simulink model "Consigna_de_torque"  (R2023b)
settings: Solver=VariableStepAuto  StartTime=0.0  StopTime=10.0  RelTol=1e-3
values from neighbouring files (symbols this model uses):
  b_eq = b_m + b_l/(r^2)    (= 2.40277777778e-05)    [definicion_cte.m]
  k_l = m*l_cm + m_l*l_l    (= 1)    [definicion_cte.m]
  L_d = 6.6e-3    (= 0.0066)    [definicion_cte.m]
  L_q = 5.8e-3    (= 0.0058)    [definicion_cte.m]
  lambda_m = 0.016    [definicion_cte.m]
  P_p = 3    [definicion_cte.m]
  r = 120    [definicion_cte.m]
settings Model: Creator=MSI  LastModifiedBy=MSI

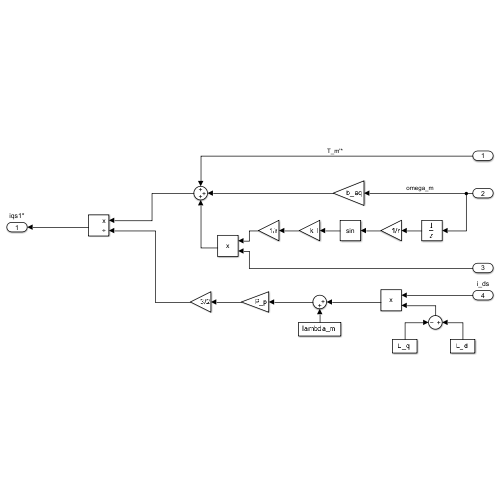
[thumbnail: Simulink's stored preview of the top-level diagram]
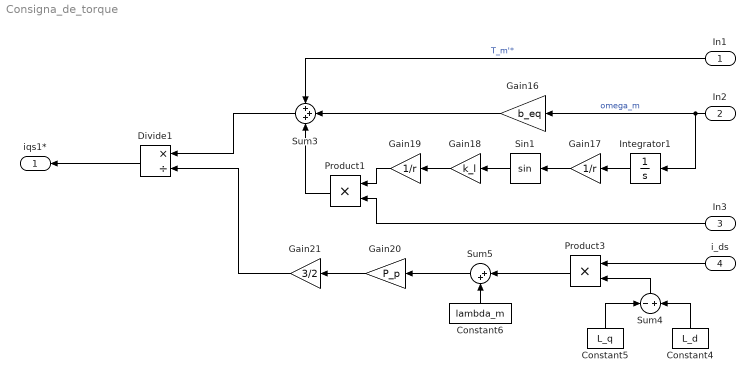
== system Consigna_de_torque ==
  In1 : Inport
  In2 : Inport  Port=2
  In3 : Inport  Port=3
  i_ds : Inport  Port=4
  Constant4 : Constant  Value=L_d
  Constant5 : Constant  Value=L_q
  Constant6 : Constant  Value=lambda_m
  Divide1 : Product  Inputs=*/
  Gain16 : Gain  Gain=b_eq
  Gain17 : Gain  Gain=1/r
  Gain18 : Gain  Gain=k_l
  Gain19 : Gain  Gain=1/r
  Gain20 : Gain  Gain=P_p
  Gain21 : Gain  Gain=3/2
  Integrator1 : Integrator
  Product1 : Product
  Product3 : Product
  Sin1 : Trigonometry
  Sum3 : Sum  Inputs=+++
  Sum4 : Sum  Inputs=-+
  Sum5 : Sum  Inputs=|++
  iqs1* : Outport
  wires:
  Gain16/1 -> Sum3/2
  In3/1 -> Product1/2
  Constant5/1 -> Sum4/1
  Gain21/1 -> Divide1/2
  Sum5/1 -> Gain20/1
  Integrator1/1 -> Gain17/1
  Gain20/1 -> Gain21/1
  Gain18/1 -> Gain19/1
  Sin1/1 -> Gain18/1
  Gain19/1 -> Product1/1
  Product1/1 -> Sum3/3
  i_ds/1 -> Product3/1
  Constant6/1 -> Sum5/2
  In1/1 -> Sum3/1  "T_m'*"
  Divide1/1 -> iqs1*/1
  Sum4/1 -> Product3/2
  Product3/1 -> Sum5/1
  Sum3/1 -> Divide1/1
  Constant4/1 -> Sum4/2
  In2/1 -> Gain16/1, Integrator1/1  "omega_m"
  Gain17/1 -> Sin1/1
